simulink model "arduino_single_motor_PWM_DIR"  (R2021b)
settings: Solver=ode4  StartTime=0.0  StopTime=inf  RelTol=1e-3  EnableMultiTasking=on
libraries: arduinolib x2, arduinosensorlib x1, simulink x1
settings Model: ExtModeTrigDuration=2  Creator=dbombara  LastModifiedBy=dbomb
settings SolverCC: AllowMultiTaskInputOutput=on  ConcurrentTasks=on
settings OptimizationCC: EnhancedBackFolding=on  PassReuseOutputArgsAs=Individual arguments  ZeroExternalMemoryAtStartup=off  ZeroInternalMemoryAtStartup=off  MaxStackSize=64  OptimizeBlockOrder=speed  DifferentSizesBufferReuse=on  OptimizationCustomize=off  EfficientTunableParamExpr=on
settings DebuggingCC: ParameterTunabilityLossMsg=error
settings HardwareCC: ProdBitPerInt=16  ProdBitPerPointer=16  ProdBitPerSizeT=16  ProdBitPerPtrDiffT=16  ProdLargestAtomicFloat=None  ProdWordSize=8  ProdHWDeviceType=Atmel->AVR
settings SFSimCC: MATLABDynamicMemAlloc=off
settings RTWCC: Description=Embedded Coder  SystemTargetFile=ert.tlc  HardwareBoard=Arduino Mega 2560  TemplateMakefile=ert_default_tmf  Toolchain=Arduino AVR  BuildConfiguration=Faster Runs
settings CodeAppCC: ForceParamTrailComments=on  IgnoreCustomStorageClasses=off  OperatorAnnotations=on  SimulinkDataObjDesc=on  SFDataObjDesc=on  InsertBlockDesc=on
settings ERTTargetCC: SupportContinuousTime=on  SupportVariableSizeSignals=on  ExtModeTransport=3  ExtModeStaticAlloc=on  ExtModeStaticAllocSize=2048  ExtModeMexFile=ext_xcp  ExtModeIntrfLevel=Level2 - Open

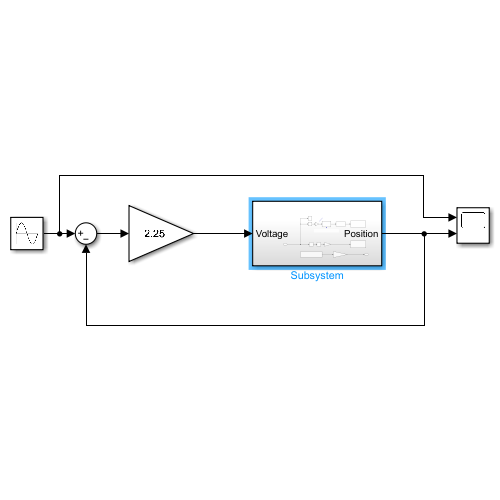
[thumbnail: Simulink's stored preview of the top-level diagram]
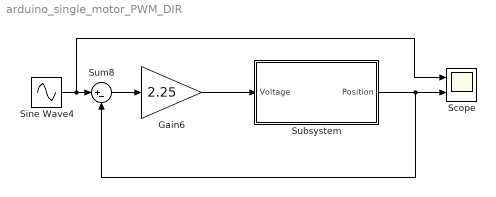
== system arduino_single_motor_PWM_DIR ==
  Gain6 : Gain  Gain=2.25
  Scope : Scope  NumInputPorts=2
  Sine Wave4 : Sin  Amplitude=10  Bias=10  Frequency=0.5  SampleTime=0
  Subsystem : Subsystem
  Sum8 : Sum  Inputs=|+-
  wires:
  Gain6/1 -> Subsystem/1(Voltage)
  Subsystem/1(Position) -> Scope/2, Sum8/2
  Sum8/1 -> Gain6/1
  Sine Wave4/1 -> Scope/1, Sum8/1

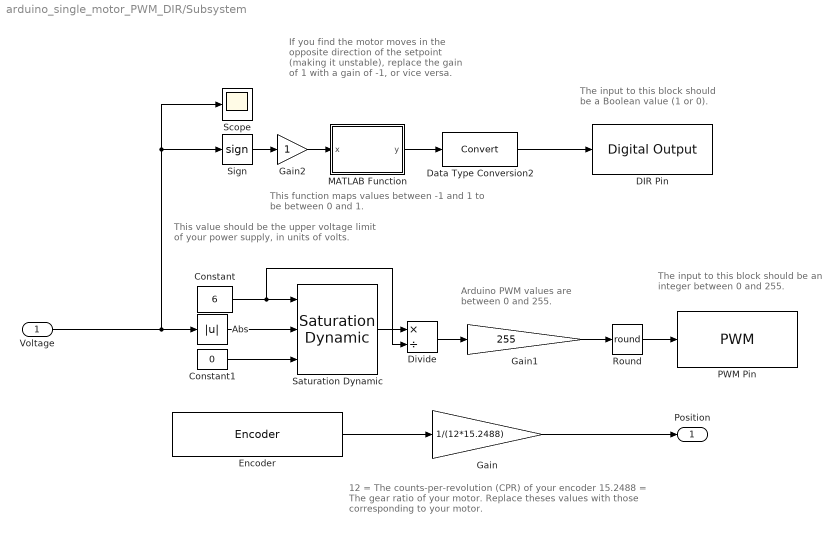
== system arduino_single_motor_PWM_DIR/Subsystem ==
  note: The input to this block should be
      | an integer between 0 and 255.
  note: The input to this block should
      | be a Boolean value (1 or 0).
  note: If you find the motor moves in the opposite direction of the setpoint (making it unstable), replace the gain of 1 with a gain of -1, or vice versa.
  note: This function maps values between -1 and 1
      | to be between 0 and 1.
  note: This value should be the upper voltage
      | limit of your power supply, in units of volts.
  note: Arduino PWM values are
      | between 0 and 255.
  note: 12 = The counts-per-revolution (CPR) of your encoder
      | 15.2488 = The gear ratio of your motor.
      | Replace theses values with those corresponding to your motor.
  Voltage : Inport
  Abs : Abs
  Constant : Constant  Value=6
  Constant1 : Constant  Value=0
  DIR Pin : arduinolib/Digital Output  pinNumber=6  Direction=output  blockPlatform=arduino
  Data Type Conversion2 : DataTypeConversion
  Divide : Product  Inputs=*/
  Encoder : arduinosensorlib/Encoder  InputA=19  InputB=18  Mode=No reset  SampleTime=-1
      settings: SourceProductBaseCode=ARDUINO
  Gain : Gain  Gain=1/(12*15.2488)
  Gain1 : Gain  Gain=255
  Gain2 : Gain
  MATLAB Function : MATLAB Function  TreatAsAtomicUnit=on
  PWM Pin : arduinolib/PWM  pinNumber=9  frequencyType=Default  desiredFrequency=1000  achievableFrequency=1000
  Round : Rounding  Operator=round
  Saturation Dynamic : simulink/Discontinuities/Saturation Dynamic  OutMin=[]  OutMax=[]  OutDataTypeStr=Inherit: Same as second input  OutDataType=fixdt(1, 16)  OutScaling=2^-10  DoSatur=off
  Scope : Scope
  Sign : Signum
  Position : Outport
  wires:
  Gain2/1 -> MATLAB Function/1(x)
  Abs/1 -> Saturation Dynamic/2
  Data Type Conversion2/1 -> DIR Pin/1
  MATLAB Function/1(y) -> Data Type Conversion2/1
  Encoder/1 -> Gain/1
  Voltage/1 -> Sign/1, Scope/1, Abs/1
  Gain/1 -> Position/1
  Sign/1 -> Gain2/1
  Saturation Dynamic/1 -> Divide/1
  Divide/1 -> Gain1/1
  Constant/1 -> Saturation Dynamic/1, Divide/2
  Constant1/1 -> Saturation Dynamic/3
  Gain1/1 -> Round/1
  Round/1 -> PWM Pin/1

== matlab function arduino_single_motor_PWM_DIR/Subsystem/MATLAB Function ==
  data: x input; y output
function y = fcn(x)
x = x*1;
y = 0.5*(x+1);
